simulink model "E2_2"  (R2022a)
settings: Solver=VariableStepAuto  StartTime=0.0  StopTime=2  MaxStep=0.001  RelTol=1e-3
InitFcn:
  | m=0.1
  | M=2
  | l=0.1
  | g=9.8
  | k=1
  | R=100
  | r=0.02
settings Model: Creator=Reza  LastModifiedBy=Reza
settings DataIOCC: ReturnWorkspaceOutputs=off

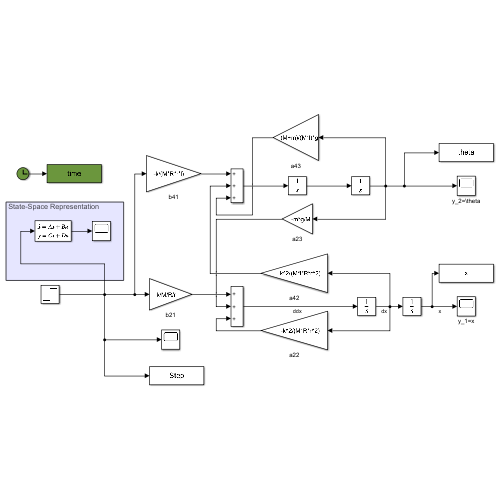
[thumbnail: Simulink's stored preview of the top-level diagram]
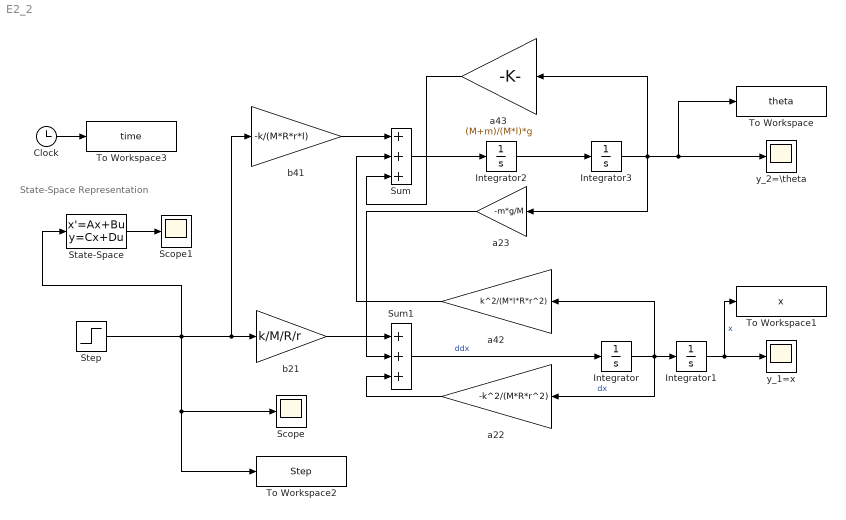
== system E2_2 ==
  note: State-Space Representation
  Clock : Clock
  Integrator{,1..3} (4 alike) : Integrator
  Scope : Scope
  Scope1 : Scope
  State-Space : StateSpace  A=[0,1,0,0;0,-k^2/(M*R*r^2),-m*g/M,0;0,0,0,1;0,k^2/(M*l*R*r^2),(M+m)/(M*l)*g,0]  B=[0;k/M/R/r;0;-k/M/l/R/r]  C=[1,0,0,0;0,0,1,0]  D=[0;0]  InitialCondition=0
  Step : Step  SampleTime=0
  Sum : Sum  Inputs=+++
  Sum1 : Sum  Inputs=+++
  To Workspace : ToWorkspace  VariableName=theta  SampleTime=-1
  To Workspace1 : ToWorkspace  VariableName=x  SampleTime=-1
  To Workspace2 : ToWorkspace  VariableName=Step  SampleTime=-1
  To Workspace3 : ToWorkspace  VariableName=time  SampleTime=-1
  a22 : Gain  Gain=-k^2/(M*R*r^2)
  a23 : Gain  Gain=-m*g/M
  a42 : Gain  Gain=k^2/(M*l*R*r^2)
  a43 : Gain  Gain=(M+m)/(M*l)*g
  b21 : Gain  Gain=k/M/R/r
  b41 : Gain  Gain=-k/(M*R*r*l)
  y_1=x : Scope
  y_2=\theta : Scope
  wires:
  a22/1 -> Sum1/3
  Integrator1/1 -> To Workspace1/1, y_1=x/1  "x"
  a42/1 -> Sum/2
  a43/1 -> Sum/3
  b21/1 -> Sum1/1
  b41/1 -> Sum/1
  Sum/1 -> Integrator2/1
  a23/1 -> Sum1/2
  Sum1/1 -> Integrator/1  "ddx"
  Integrator2/1 -> Integrator3/1
  Step/1 -> State-Space/1, To Workspace2/1, Scope/1, b21/1, b41/1
  Integrator3/1 -> a43/1, To Workspace/1, y_2=\theta/1, a23/1
  Integrator/1 -> Integrator1/1, a42/1, a22/1  "dx"
  State-Space/1 -> Scope1/1
  Clock/1 -> To Workspace3/1
